simulink model "Enceinte_climatique_2"  (R2025b)
settings: Solver=VariableStepAuto  StartTime=0.0  StopTime=10.0  RelTol=1e-3
settings Model: Creator=rofte  LastModifiedBy=rofte

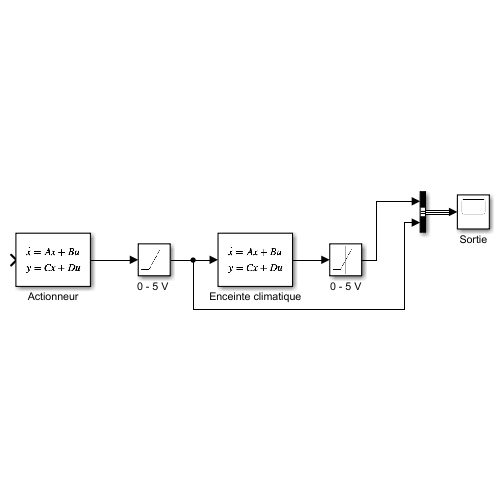
[thumbnail: Simulink's stored preview of the top-level diagram]
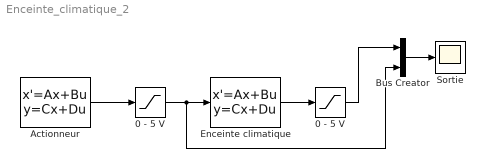
== system Enceinte_climatique_2 ==
  0 - 5 V : Saturate  UpperLimit=5  LowerLimit=0  LinearizeAsGain=off
  "0 - 5 V " : Saturate  UpperLimit=5  LowerLimit=0
  Actionneur : StateSpace  A=-2  B=60  D=0  InitialCondition=0
  Bus Creator : BusCreator  Inputs=2
  Enceinte climatique : StateSpace  A=-2  B=2  D=0  InitialCondition=0
  Sortie : Scope
      settings: ActiveDisplayYMinimum=-3.644200174510388  ActiveDisplayYMaximum=5.9014912360284031
  wires:
  Enceinte climatique/1 -> 0 - 5 V/1
  Bus Creator/1 -> Sortie/1
  "0 - 5 V "/1 -> Bus Creator/2, Enceinte climatique/1
  0 - 5 V/1 -> Bus Creator/1
  Actionneur/1 -> "0 - 5 V "/1
